simulink model "gpsTestHarness"  (R2024a)
settings: configuration reference "standardSILConfiguraitonParams" (kept outside this file)
undefined symbols (not defined in the file): referenceLatitude_deg, referenceLongitude_deg, terrainHeightNED_m
settings Model: Creator=aeroth  LastModifiedBy=jerem
settings ConfigSetRef: SourceName=standardSILConfiguraitonParams  SourceLocation=Base Workspace

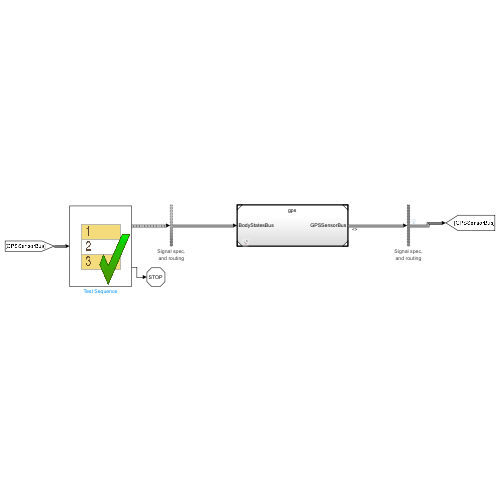
[thumbnail: Simulink's stored preview of the top-level diagram]
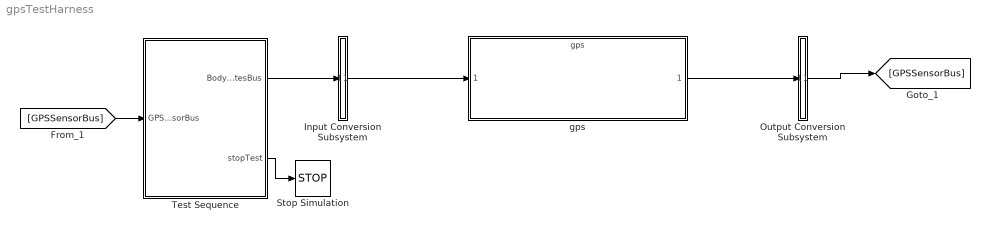
== system gpsTestHarness ==
  Input Conversion Subsystem : Subsystem  Tag=__SLT_ICS__  Description=|
      | Signal spec.
      | and routing
      settings: AttributesFormatString=%<Description>
  Output Conversion Subsystem : Subsystem  Tag=__SLT_OCS__  Description=|
      | Signal spec.
      | and routing
      mask init:
      | ICDictionary = get_param(bdroot, 'DataDictionary');
      | if isempty(ICDictionary)
      |    ICScope = Simulink.data.BaseWorkspace;
      | else
      |    ICScope = Simulink.data.DataDictionary(ICDictionary);
      | end
      | 
      | IC1 = Simulink.Bus.createMATLABStruct('GPSSensorBus', [], [1 1], ICScope);
      settings: AttributesFormatString=%<Description>
  Stop Simulation : Stop
  Test Sequence : Test Sequence  TreatAsAtomicUnit=on
  gps : ModelReference  ModelNameDialog=gps  SimulationMode=Normal  ModelReferenceVersion=1.43
  wires:
  Test Sequence/1(BodyStatesBus) -> Input Conversion Subsystem/1(Inport_1)
  [GPSSensorBus] -> Test Sequence/1(GPSSensorBus)
  Output Conversion Subsystem/1(Outport_1) -> [GPSSensorBus]
  Test Sequence/2(stopTest) -> Stop Simulation/1
  gps/1 -> Output Conversion Subsystem/1(Inport_1)
  Input Conversion Subsystem/1(Outport_1) -> gps/1

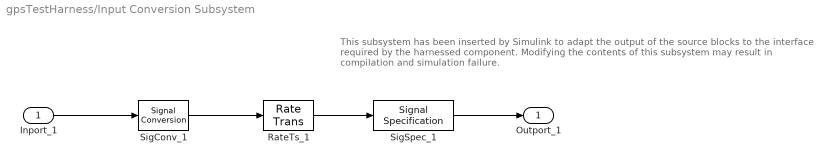
== system gpsTestHarness/Input Conversion Subsystem ==
  note: This subsystem has been inserted by Simulink to adapt the output of the source blocks to the interface required by the harnessed component.
      |  Modifying the contents of this subsystem may result in compilation and simulation failure.
  Inport_1 : Inport
  RateTs_1 : RateTransition  OutPortSampleTime=0.004
  SigConv_1 : SignalConversion  ConversionOutput=Virtual bus  OverrideOpt=off
  SigSpec_1 : SignalSpecification  OutDataTypeStr=Bus: BodyStateBus  SampleTime=0.004
  Outport_1 : Outport
  wires:
  SigSpec_1/1 -> Outport_1/1
  RateTs_1/1 -> SigSpec_1/1
  SigConv_1/1 -> RateTs_1/1
  Inport_1/1 -> SigConv_1/1

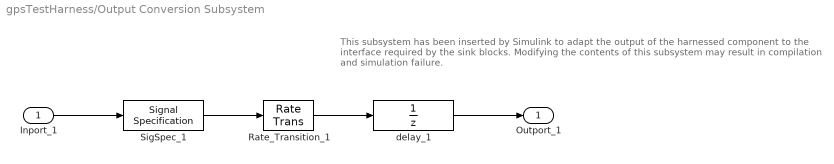
== system gpsTestHarness/Output Conversion Subsystem ==
  note: This subsystem has been inserted by Simulink to adapt the output of the harnessed component to the interface required by the sink blocks.
      |  Modifying the contents of this subsystem may result in compilation and simulation failure.
  Inport_1 : Inport
  Rate_Transition_1 : RateTransition  OutPortSampleTimeOpt=Inherit
  SigSpec_1 : SignalSpecification  OutDataTypeStr=Bus: GPSSensorBus  Dimensions=[1]  SampleTime=0.004
  delay_1 : UnitDelay  InitialCondition=IC1  SampleTime=-1
  Outport_1 : Outport
  wires:
  Inport_1/1 -> SigSpec_1/1
  SigSpec_1/1 -> Rate_Transition_1/1
  Rate_Transition_1/1 -> delay_1/1
  delay_1/1 -> Outport_1/1

== stateflow chart gpsTestHarness/Test Sequence ==
  state Scenario_1
    state Initialize
      %% Initialize data outputs.
      stopTest = false;
      BodyStatesBus.aircraftVelInNED_mps = zeros(3,1);
      BodyStatesBus.aircraftPosInNED_m = zeros(3,1);
      BodyStatesBus.aircraftEulerAngles_rad = zeros(3,1);
      BodyStatesBus.aircraftVelInBody_mps = zeros(3,1);
      BodyStatesBus.aircraftAngVelInBody_radps = zeros(3,1);
      BodyStatesBus.aircraftAngAccelInBody_radps2 = zeros(3,1);
      BodyStatesBus.aircraftAccelInBody_mps2 = zeros(3,1);
      BodyStatesBus.DCM_be = zeros(3,3);
    state checkGpsStatic
      verify(isClose(GPSSensorBus.lat_deg, referenceLatitude_deg))
      verify(isClose(GPSSensorBus.lon_deg, referenceLongitude_deg))
      verify(isClose(GPSSensorBus.alt_m, terrainHeightNED_m, 'atol', 0.5))
      verify(isClose(GPSSensorBus.vel_mps, 0, 'atol', 0.5))
      verify(isClose(GPSSensorBus.vel_n_mps, 0, 'atol', 0.5))
      verify(isClose(GPSSensorBus.vel_e_mps, 0, 'atol', 0.5))
      verify(isClose(GPSSensorBus.vel_d_mps, 0, 'atol', 0.5))
    state goHighDynamic
      BodyStatesBus.aircraftVelInNED_mps = [10 20 30]';
      BodyStatesBus.aircraftPosInNED_m = [0 0 -3048]';
      BodyStatesBus.aircraftEulerAngles_rad = [0.1 0.2 0.3]';
      BodyStatesBus.aircraftVelInBody_mps = zeros(3,1);
      BodyStatesBus.aircraftAngVelInBody_radps =  [0.1 0.2 0.3]';
      BodyStatesBus.aircraftAngAccelInBody_radps2 =  [0.1 0.2 0.3]';
      BodyStatesBus.aircraftAccelInBody_mps2 =  [0.1 0.2 0.3]';
      BodyStatesBus.DCM_be = zeros(3,3);
    state checkHighDynamic
      verify(isClose(GPSSensorBus.lat_deg, referenceLatitude_deg))
      verify(isClose(GPSSensorBus.lon_deg, referenceLongitude_deg))
      verify(isClose(GPSSensorBus.alt_m, 3048 + terrainHeightNED_m))
      verify(isClose(GPSSensorBus.vel_mps, norm([10 20 30]), 'rtol', 0.8)) %why is this one so bad?
      verify(isClose(GPSSensorBus.vel_n_mps, 10, 'rtol', 0.1))
      verify(isClose(GPSSensorBus.vel_e_mps, 20, 'rtol', 0.1))
      verify(isClose(GPSSensorBus.vel_d_mps, 30, 'rtol', 0.1))
    state EndTest
      stopTest = true;
    (default) -> Initialize
    Initialize -> checkGpsStatic : [
        | true
        | ]
    checkGpsStatic -> goHighDynamic : [
        | true
        | ]
    goHighDynamic -> checkHighDynamic : [
        | true
        | ]
    checkHighDynamic -> EndTest : [
        | true
        | ]
  (default) -> Scenario_1 : {assert(Active_Scenario_Index == 1,'The value of Scenario Parameter ''Active_Scenario_Index'' is not valid. Use the index of the scenario to specify it.')}
  data: GPSSensorBus input Bus: GPSSensorBus size=[1]; BodyStatesBus output Bus: BodyStateBus size=[1]; Active_Scenario_Index parameter =1; stopTest output; referenceLatitude_deg parameter; referenceLongitude_deg parameter; terrainHeightNED_m parameter
